simulink model "dynamic_off_D"  (R2015b)
settings: Solver=VariableStepAuto  StartTime=0.0  StopTime=5  RelTol=1e-3
libraries: powerlib x17, powerlib_extras x5, powerlib_meascontrol x1
settings Model: Creator=fujitsu  LastModifiedBy=fujitsu

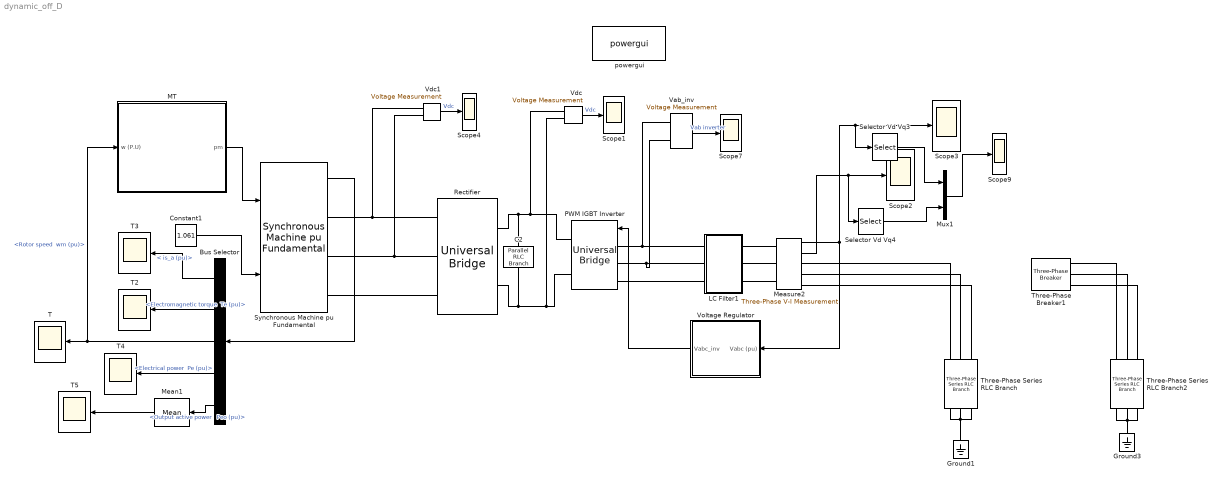
== system dynamic_off_D ==
  Bus Selector : BusSelector  OutputSignals="Stator current. is_a (pu),Mechanical.Electromagnetic torque  Te (pu),Mechanical.Rotor speed  wm (pu),Mechanical.Electrical power  Pe (pu),Output active power   Peo (pu)"
  C2 : powerlib/Elements/Parallel RLC Branch  LConnTagsString=a  RConnTagsString=__new0  BranchType=C  Resistance=inf  Inductance=inf  SetiL0=off  InitialCurrent=0  Capacitance=5000e-06  Setx0=off  InitialVoltage=0  Measurements=None
  Constant1 : Constant  Value=1.061
  Ground1 : powerlib/Elements/Ground  LConnTagsString=a
  Ground3 : powerlib/Elements/Ground  LConnTagsString=a
  LC Filter1 : Subsystem
  MT : Subsystem
  Mean1 : powerlib_meascontrol/Measurements/Mean  Freq=50  Vinit=0  Ts=50e-6
  Measure2 : powerlib/Measurements/Three-Phase V-I Measurement  VoltageMeasurement=phase-to-phase  SetLabelV=off  LabelV=V1  Vpu=off  VpuLL=on  CurrentMeasurement=yes  SetLabelI=off  LabelI=I1  Ipu=on  Pbase=10e3  Vbase=400  OutputType=Magnitude  PhasorSimulation=off  PSBequivalent=0
  Mux1 : Mux  Inputs=2
  PWM IGBT Inverter : powerlib/Power Electronics/Universal Bridge  Arms=3  SnubberResistance=5000  SnubberCapacitance=inf  Device=IGBT / Diodes  Ron=1e-3  Lon=0  ForwardVoltages="[  0.0  0.0  ]"  ForwardVoltage=.8  GTOparameters=[ 1e-6 ,1e-6 ]  IGBTparameters=[ 1e-6 , 2e-6 ]  Measurements=Device currents  Measurements_2=None  converterType=Rectifier
  Rectifier : powerlib/Power Electronics/Universal Bridge  Arms=3  SnubberResistance=50  SnubberCapacitance=0.1e-6  Device=Diodes  Ron=1e-3  Lon=0  ForwardVoltages="[  0.8  0.8  ]"  ForwardVoltage=.7  GTOparameters=[ 10e-6 , 20e-6 ]  IGBTparameters=[ 1e-6 , 2e-6 ]  Measurements=Device currents  Measurements_2=None  converterType=Rectifier
  Scope{1..4,7,9} (6 alike) : Scope
  Selector Vd Vq3 : Selector  InputPortWidth=3  IndexOptions=Index vector (dialog)  Indices=[1]  OutputSizes=1
  Selector Vd Vq4 : Selector  InputPortWidth=3  IndexOptions=Index vector (dialog)  Indices=[1]  OutputSizes=1
  Synchronous Machine pu Fundamental : powerlib/Machines/Synchronous Machine pu Fundamental  PresetModel=No  MechanicalLoad=Mechanical power Pm  ShowDetailedParameters=on  RotorType=Salient-pole  Units=per unit fundamental parameters  MeasurementBus=off  NominalParameters="[ 65e3  500 1600]"  Stator="[ 0.2503  0.114  0.6875  0.6875 ]"  Field="[ 1  10e15/(100*pi)]"  Dampers2=[0.0652, 0.5134, 0.0287, 0.2553, 7.765e-3, 0.9167 ]  Dampers1="[ 1.17E-02  0.182  1.97E-02  0.384 ]"  Mechanical=[ 6 0 2]  PolePairs=20  InitialConditions="[ 0  0  0  0  0  0  0  0  1 ]"  SetSaturation=off  Saturation=[0.6404,0.7127,0.8441,0.9214,0.9956,1.082,1.19,1.316,1.457;0.7,0.7698,0.8872,0.9466,0.9969,1.046,1.1,1.151,1.201]  LoadFlowParameters=[1,0,0,0,0]  TsPowergui=0  TsBlock=-1  IterativeModel=Trapezoidal non iterative  BusType=swing  Pref=0  Qref=0  Qmin=-inf  Qmax=inf  PLF=0  QLF=0
  T{,2..5} (5 alike) : Scope
  Three-Phase Series RLC Branch : powerlib/Elements/Three-Phase Series RLC Branch  LConnTagsString=A|B|C  RConnTagsString=A|B|C  BranchType=R  Resistance=50  Inductance=1e-3  Capacitance=1e-6  Measurements=None
  Three-Phase Series RLC Branch2 : powerlib/Elements/Three-Phase Series RLC Branch  LConnTagsString=A|B|C  RConnTagsString=A|B|C  BranchType=R  Resistance=50  Inductance=1e-3  Capacitance=1e-6  Measurements=None
  Three-Phase Breaker1 : powerlib/Elements/Three-Phase Breaker  InitialState=open  SwitchA=on  SwitchB=on  SwitchC=on  SwitchTimes=[2.5]  External=off  BreakerResistance=0.01  SnubberResistance=1e6  SnubberCapacitance=inf  Measurements=None
  Vab_inv : powerlib/Measurements/Voltage Measurement  Tag=PoWeRsYsTeMmEaSuReMeNt  PhasorSimulation=off  OutputType=Magnitude  PSBequivalent=0
  Vdc : powerlib/Measurements/Voltage Measurement  Tag=PoWeRsYsTeMmEaSuReMeNt  PhasorSimulation=off  OutputType=Magnitude  PSBequivalent=0
  Vdc1 : powerlib/Measurements/Voltage Measurement  Tag=PoWeRsYsTeMmEaSuReMeNt  PhasorSimulation=off  OutputType=Magnitude  PSBequivalent=0
  Voltage Regulator : Subsystem  mask{kp=0.01, ki=5}
  powergui : powerlib/powergui  SimulationMode=Discrete  SolverType=Tustin  SampleTime=5e-6  frequency=60  SPID=off  DisableSnubberDevices=off  DisableRonSwitches=off  DisableVfSwitches=off  SwTol=0  DisplayEquations=off  Interpol=off  ExternalGateDelay=off  methode=off  Ts=0  FunctionMessages=off  echomessages=off  HookPort=off  EnableUseOfTLC=off  x0status=blocks  frequencyindice=0  Pbase=100e6  ErrMax=0.0001  Iterations=50  UnitsV=kV  UnitsW=MW  buscounter=0  RestoreLinks=warning  ResistiveCurrentMeasurement=off  Frange=[0:2:500]  Ylog=off  Xlog=on  ShowGrid=off  save=off  variable=ZData  structure=Vs  ZoomFFT=on  StartTime=1/60  cycles=1  DisplayStyle=1  fundamental=60  FreqAxis=on  MaxFrequency=10000  frequencyindicesteady=1  RmsSteady=1  display=off
  wires:
  Vdc/1 -> Scope1/1  "Vdc"
  Vab_inv/1 -> Scope7/1  "Vab inverter"
  Voltage Regulator/1(Vabc_inv) -> PWM IGBT Inverter/1
  Measure2/1 -> Voltage Regulator/1(Vabc (pu)), Selector Vd Vq3/1, Scope3/1
  Vdc1/1 -> Scope4/1  "Vdc"
  Measure2/2 -> Selector Vd Vq4/1, Scope2/1
  Mux1/1 -> Scope9/1
  Selector Vd Vq3/1 -> Mux1/1
  Selector Vd Vq4/1 -> Mux1/2
  Synchronous Machine pu Fundamental/1 -> Bus Selector/1
  Bus Selector/1 -> T3/1  "< is_a (pu)>"
  Bus Selector/2 -> T2/1  "<Electromagnetic torque  Te (pu)>"
  Bus Selector/3 -> MT/1(w (P.U)), T/1  "<Rotor speed  wm (pu)>"
  Constant1/1 -> Synchronous Machine pu Fundamental/2
  Bus Selector/4 -> T4/1  "<Electrical power  Pe (pu)>"
  Bus Selector/5 -> Mean1/1  "<Output active power   Peo (pu)>"
  Mean1/1 -> T5/1
  MT/1(pm) -> Synchronous Machine pu Fundamental/1
  connections:
  C2/LConn1 -- Rectifier/RConn1 -- PWM IGBT Inverter/RConn1 -- Vdc/LConn1
  Measure2/RConn1 -- Three-Phase Series RLC Branch/LConn1
  Rectifier/RConn2 -- C2/RConn1 -- PWM IGBT Inverter/RConn2 -- Vdc/LConn2
  Measure2/RConn2 -- Three-Phase Series RLC Branch/LConn2
  Vdc1/LConn1 -- Rectifier/LConn1 -- Synchronous Machine pu Fundamental/RConn1
  Vdc1/LConn2 -- Rectifier/LConn2 -- Synchronous Machine pu Fundamental/RConn2
  Three-Phase Series RLC Branch/RConn2 -- Ground1/LConn1 -- Three-Phase Series RLC Branch/RConn3 -- Three-Phase Series RLC Branch/RConn1
  Three-Phase Series RLC Branch/LConn3 -- Measure2/RConn3
  LC Filter1/RConn1 -- Measure2/LConn1
  LC Filter1/RConn2 -- Measure2/LConn2
  LC Filter1/RConn3 -- Measure2/LConn3
  Vab_inv/LConn1 -- LC Filter1/LConn1 -- PWM IGBT Inverter/LConn1
  PWM IGBT Inverter/LConn2 -- Vab_inv/LConn2 -- LC Filter1/LConn2
  PWM IGBT Inverter/LConn3 -- LC Filter1/LConn3
  Synchronous Machine pu Fundamental/RConn3 -- Rectifier/LConn3
  Three-Phase Series RLC Branch2/RConn2 -- Three-Phase Series RLC Branch2/RConn3 -- Ground3/LConn1 -- Three-Phase Series RLC Branch2/RConn1
  Three-Phase Breaker1/RConn3 -- Three-Phase Series RLC Branch2/LConn3
  Three-Phase Breaker1/RConn2 -- Three-Phase Series RLC Branch2/LConn2
  Three-Phase Breaker1/RConn1 -- Three-Phase Series RLC Branch2/LConn1

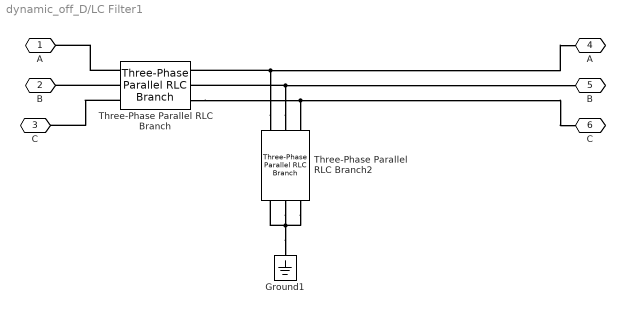
== system dynamic_off_D/LC Filter1 ==
  Ground1 : powerlib/Elements/Ground  LConnTagsString=a
  Three-Phase Parallel RLC Branch : powerlib/Elements/Three-Phase Parallel RLC Branch  LConnTagsString=A|B|C  RConnTagsString=A|B|C  BranchType=L  Resistance=1  Inductance=5.7e-3  Capacitance=1e-6  Measurements=None
  Three-Phase Parallel RLC Branch2 : powerlib/Elements/Three-Phase Parallel RLC Branch  LConnTagsString=A|B|C  RConnTagsString=A|B|C  BranchType=C  Resistance=1  Inductance=5.7e-3  Capacitance=1000e-6  Measurements=None
  A : PMIOPort  Port=1  Side=Left
  B : PMIOPort  Port=2  Side=Left
  C : PMIOPort  Port=3  Side=Left
  "A " : PMIOPort  Port=4  Side=Right
  "B " : PMIOPort  Port=5  Side=Right
  "C " : PMIOPort  Port=6  Side=Right
  connections:
  Ground1/LConn1 -- Three-Phase Parallel RLC Branch2/RConn2 -- Three-Phase Parallel RLC Branch2/RConn1 -- Three-Phase Parallel RLC Branch2/RConn3
  Three-Phase Parallel RLC Branch/RConn3 -- Three-Phase Parallel RLC Branch2/LConn3 -- "C "/RConn1
  Three-Phase Parallel RLC Branch2/LConn2 -- "B "/RConn1 -- Three-Phase Parallel RLC Branch/RConn2
  Three-Phase Parallel RLC Branch2/LConn1 -- "A "/RConn1 -- Three-Phase Parallel RLC Branch/RConn1
  Three-Phase Parallel RLC Branch/LConn3 -- C/RConn1
  Three-Phase Parallel RLC Branch/LConn2 -- B/RConn1
  Three-Phase Parallel RLC Branch/LConn1 -- A/RConn1

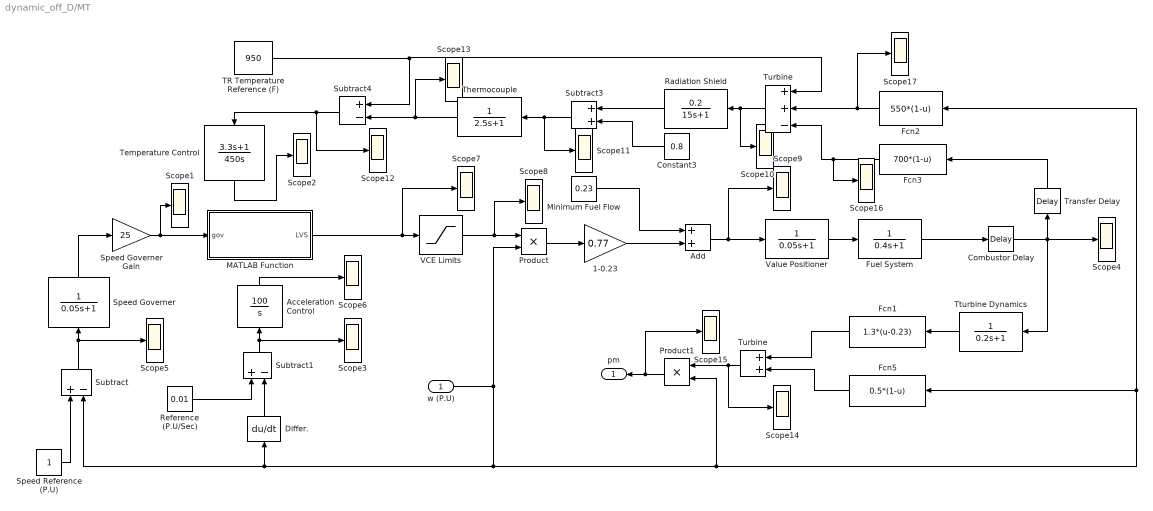
== system dynamic_off_D/MT ==
  w (P.U) : Inport
  1-0.23 : Gain  Gain=0.77
  Acceleration Control : TransferFcn  Numerator=[0 100]  Denominator=[1 0]
  Add : Sum
  Combustor Delay : TransportDelay  DelayTime=0.01
  Constant3 : Constant  Value=0.8
  Differ. : Derivative
  Fcn1 : Fcn  Expr=1.3*(u-0.23)
  Fcn2 : Fcn  Expr=550*(1-u)
  Fcn3 : Fcn  Expr=700*(1-u)
  Fcn5 : Fcn  Expr=0.5*(1-u)
  Fuel System : TransferFcn  Denominator=[0.4 1]
  MATLAB Function : MATLAB Function  TreatAsAtomicUnit=on
  Minimum Fuel Flow : Constant  Value=0.23
  Product : Product  RndMeth=Zero
  Product1 : Product  RndMeth=Zero
  Radiation Shield : TransferFcn  Numerator=[0.2]  Denominator=[15 1]
  Reference (P.U/Sec) : Constant  Value=0.01
  Scope{1..17} (17 alike) : Scope
  Speed Governer : TransferFcn  Denominator=[0.05 1]
  Speed Governer Gain : Gain  Gain=25
  Speed Reference (P.U) : Constant
  Subtract : Sum  Inputs=+-
  Subtract1 : Sum  Inputs=+-
  Subtract3 : Sum
  Subtract4 : Sum  Inputs=+-
  TR Temperature Reference (F) : Constant  Value=950
  Temperature Control : TransferFcn  Numerator=[3.3 1]  Denominator=[450 0]
  Thermocouple : TransferFcn  Denominator=[2.5 1]
  Transfer Delay : TransportDelay  DelayTime=0.04
  Tturbine Dynamics : TransferFcn  Denominator=[0.2 1]
  Turbine : Sum  Inputs=++-
  "Turbine " : Sum
  VCE Limits : Saturate  UpperLimit=1.5  LowerLimit=-0.1
  Value Positioner : TransferFcn  Denominator=[0.05 1]
  pm : Outport
  wires:
  Speed Reference (P.U)/1 -> Subtract/1
  Subtract/1 -> Scope5/1, Speed Governer/1
  VCE Limits/1 -> Scope8/1, Product/1
  Product/1 -> 1-0.23/1
  1-0.23/1 -> Add/2
  Minimum Fuel Flow/1 -> Add/1
  Add/1 -> Scope9/1, Value Positioner/1
  Value Positioner/1 -> Fuel System/1
  Fuel System/1 -> Combustor Delay/1
  Combustor Delay/1 -> Scope4/1, Tturbine Dynamics/1, Transfer Delay/1
  Speed Governer Gain/1 -> Scope1/1, MATLAB Function/1(gov)
  Differ./1 -> Subtract1/2
  Reference (P.U/Sec)/1 -> Subtract1/1
  Subtract1/1 -> Scope3/1, Acceleration Control/1
  Acceleration Control/1 -> Scope6/1
  Transfer Delay/1 -> Fcn3/1
  Fcn3/1 -> Scope16/1, Turbine/3
  Fcn2/1 -> Scope17/1, Turbine/2
  Radiation Shield/1 -> Subtract3/1
  Constant3/1 -> Subtract3/2
  Turbine/1 -> Scope10/1, Radiation Shield/1
  Subtract3/1 -> Scope11/1, Thermocouple/1
  Thermocouple/1 -> Scope13/1, Subtract4/2
  TR Temperature Reference (F)/1 -> Turbine/1, Subtract4/1
  Subtract4/1 -> Scope12/1, Temperature Control/1
  Temperature Control/1 -> Scope2/1
  Speed Governer/1 -> Speed Governer Gain/1
  w (P.U)/1 -> Product/2, Subtract/2, Differ./1, Product1/2, Fcn5/1, Fcn2/1
  Tturbine Dynamics/1 -> Fcn1/1
  Fcn1/1 -> "Turbine "/1
  Fcn5/1 -> "Turbine "/2
  Product1/1 -> Scope15/1, pm/1
  "Turbine "/1 -> Scope14/1, Product1/1
  MATLAB Function/1(LVS) -> Scope7/1, VCE Limits/1

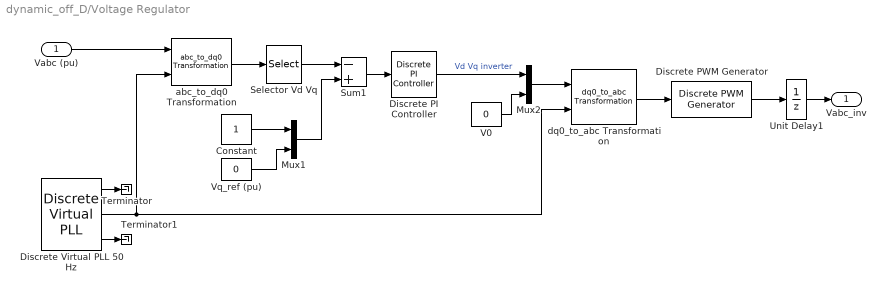
== system dynamic_off_D/Voltage Regulator ==
  Vabc (pu) : Inport
  Constant : Constant
  Discrete PI Controller : powerlib_extras/Discrete  Control Blocks/Discrete PI Controller  Kp=kp  Ki=ki  Par_Limits=[1 -1]  Init=0  Ts=5e-6
  Discrete PWM Generator : powerlib_extras/Discrete  Control Blocks/Discrete PWM Generator  GeneratorMode="3-arm  bridge (6 pulses)"  Fc=2000  Ts=5e-6  Internal=off  mIndex=0.4  Freq=60  Phase=0
  Discrete Virtual PLL 50 Hz : powerlib_extras/Discrete  Control Blocks/Discrete Virtual PLL  Freq=50  Phase=0  Ts=5e-6
  Mux1 : Mux  Inputs=2
  Mux2 : Mux  Inputs=2
  Selector Vd Vq : Selector  InputPortWidth=3  IndexOptions=Index vector (dialog)  Indices=[1 2]  OutputSizes=1
  Sum1 : Sum  Inputs=-+  SaturateOnIntegerOverflow=on  InputSameDT=on  OutDataTypeStr=Inherit: Same as first input
  Terminator : Terminator
  Terminator1 : Terminator
  Unit Delay1 : UnitDelay  SampleTime=2e-6
  V0 : Constant  Value=0
  Vq_ref (pu) : Constant  Value=0
  abc_to_dq0 Transformation : powerlib_extras/Measurements/abc_to_dq0 Transformation
  dq0_to_abc Transformation : powerlib_extras/Measurements/dq0_to_abc Transformation
  Vabc_inv : Outport
  wires:
  abc_to_dq0 Transformation/1 -> Selector Vd Vq/1
  Vabc (pu)/1 -> abc_to_dq0 Transformation/1
  Selector Vd Vq/1 -> Sum1/1
  Sum1/1 -> Discrete PI Controller/1
  Mux2/1 -> dq0_to_abc Transformation/1
  V0/1 -> Mux2/2
  Discrete Virtual PLL 50 Hz/2 -> abc_to_dq0 Transformation/2, dq0_to_abc Transformation/2
  Constant/1 -> Mux1/1
  Vq_ref (pu)/1 -> Mux1/2
  Mux1/1 -> Sum1/2
  Discrete Virtual PLL 50 Hz/1 -> Terminator/1
  Discrete Virtual PLL 50 Hz/3 -> Terminator1/1
  Discrete PI Controller/1 -> Mux2/1  "Vd Vq inverter"
  Discrete PWM Generator/1 -> Unit Delay1/1
  dq0_to_abc Transformation/1 -> Discrete PWM Generator/1
  Unit Delay1/1 -> Vabc_inv/1

== matlab function dynamic_off_D/MT/MATLAB Function ==
  data: gov input; LVS output
function LVS= MT(gov)
T=1000e-6;
wref=1;
W=25;
X=0;
Y=0.05;
Z=1;
a1=wref-0.985;
a2=wref-0.986;
a3=wref-0.987;
a4=wref-0.988;
a5=wref-0.989;
a6=wref-0.990;
a7=wref-0.991;
a8=wref-0.992;
a9=wref-0.993;
a10=wref-0.994;
a11=wref-0.995;
a12=wref-0.996;
a13=wref-0.997;
a14=wref-0.998;
a15=wref-0.999;
a16=wref-1;
a17=wref-1.001;
a18=wref-1.002;
a19=wref-1.003;
a20=wref-1.004;
a21=wref-1.005;
a=[a1 a2 a3 a4 a5 a6 a7 a8 a9 a10 a11 a12 a13 a14 a15 a16 a17 a18 a19 a20 a21];
g=zeros(1,21);
for i=1:21
    A=a(i);
  gov=(W*T*A)/Y+gov*(1-(Z*T)/Y);
  g(i)=gov;
end
[y,x]=min(g);
LVS=y;
